simulink model "SIGNAL2"  (R2020a)
settings: Solver=VariableStepAuto  StartTime=0.0  StopTime=10.0  RelTol=1e-3
libraries: simulink x1
settings Model: Creator=86150  LastModifiedBy=86150

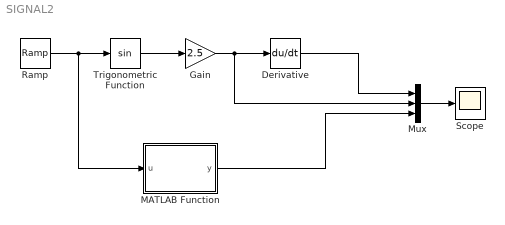
== system SIGNAL2 ==
  Derivative : Derivative
  Gain : Gain  Gain=2.5
  MATLAB Function : MATLAB Function  TreatAsAtomicUnit=on
  Mux : Mux  Inputs=3
  Ramp : simulink/Sources/Ramp  slope=1  start=0  InitialOutput=0  VectorParams1D=off
  Scope : Scope
  Trigonometric Function : Trigonometry
  wires:
  Derivative/1 -> Mux/1
  Trigonometric Function/1 -> Gain/1
  Gain/1 -> Derivative/1, Mux/2
  Ramp/1 -> MATLAB Function/1(u), Trigonometric Function/1
  Mux/1 -> Scope/1
  MATLAB Function/1(y) -> Mux/3

== matlab function SIGNAL2/MATLAB Function ==
  data: u input; y output
function y = fcn(u)

y = sin(u-pi/4);
